simulink model "Playground"  (R2022a)
settings: Solver=VariableStepAuto  StartTime=0.0  StopTime=10.0  RelTol=1e-3
undefined symbols (not defined in the file): canChannel
libraries: canlib x4, canmsglib x2
settings Model: Creator=maxju  LastModifiedBy=maxju

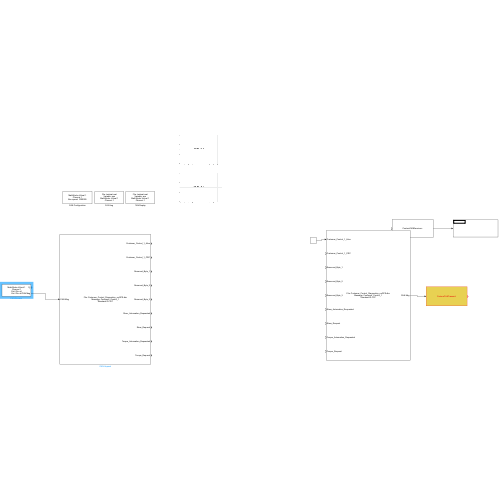
[thumbnail: Simulink's stored preview of the top-level diagram]
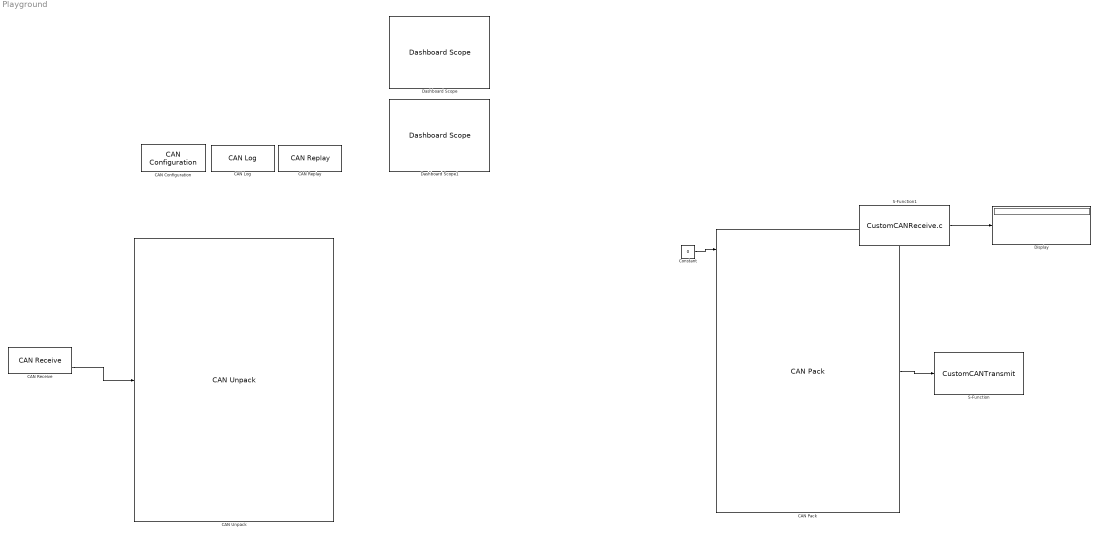
== system Playground ==
  CAN Configuration : canlib/CAN Configuration  BlockHandle=701.0001  Device=MathWorks Virtual 1 (Channel 1)  DeviceMenu=MathWorks Virtual 1 (Channel 1)  ObjConstructor=canChannel('MathWorks', 'Virtual 1', 1)  BusSpeed=1000000  EnableBitParameters=off  AckMode=Normal
      settings: SourceProductBaseCode=VN
  CAN Log : canlib/CAN Log  BlockHandle=706.0004  FullPathFileName=C:\Workspace\MATLAB Scripts\CAN_Blocks\testmat.mat  FileName=testmat.mat  VariableName=ans  MaxNumMessages=10000  LogFrom=CAN Bus  DeviceMenu=MathWorks Virtual 1 (Channel 1)  Device=MathWorks Virtual 1 (Channel 1)  ObjConstructor=canChannel('MathWorks', 'Virtual 1', 1)  SampleTime=0.01
      settings: SourceProductBaseCode=VN
  CAN Pack : canmsglib/CAN Pack  CANdbFile=C:\Workspace\XCU_eNV200_Shiftec\CAN\Customer_Control_Diagnostics_noGPS.dbc  MsgList=Customer_Control_1  MsgName=Customer_Control_1  MsgIDType=Standard (11-bit identifier)  MsgIdentifier=257  MsgLength=8  Remote=off  ApplyMinMax=off  BusOutput=off  SignalInfo={'Customer_Control_1_Alive','8','8','LE','unsigned','Standard','0','1','0','0','255';'Customer_Control_1_CRC','0','8','LE','unsigned','Standard','0','1','0','0','255';'Reserved_Byte_1','32','8','LE','unsigned','Standard','0','1','0','0','255';'Reserved_Byte_2','40','8','LE','unsigned','Standard','0','1','0','0','255';'Reserved_Byte_3','48','8','LE','unsigned','Standard','0','1','0','0','255';'Steer_Automation_Requested','56','1','LE','unsigned','Standard','0','1','0','0','1';'Steer_Request','16','8','LE','signed','Standard','0','1','0','-100','100';'Torque_Automation_Requested','60','1','LE','unsigned','Standard','0','1','0','0','1';'Torque_Request','24','8','LE','signed','Standard','0','1','0','-100','100'}
      settings: SourceProductBaseCode=XP,ME,VN  DataFormat=CANdb specified signals
  CAN Receive : canlib/CAN Receive  BlockHandle=702.0004  Device=MathWorks Virtual 1 (Channel 1)  DeviceMenu=MathWorks Virtual 1 (Channel 1)  ObjConstructor=canChannel('MathWorks', 'Virtual 1', 1)  EnableStandardIDsFilter=off  StdIDsCombo=Allow all  StandardIDs=0  EnableExtendedIDsFilter=off  ExtIDsCombo=Allow all  ExtendedIDs=0  SampleTime=0.01  MsgsPerTimestep=all  InternalFilterUpdateStatus=on  BusOutput=off
      settings: SourceProductBaseCode=VN
  CAN Replay : canlib/CAN Replay  BlockHandle=705.0002  FullPathFileName=C:\Workspace\MATLAB Scripts\CAN_Blocks\testmat.mat  FileName=testmat.mat  VariableName=ans  NoTimesReplay=Inf  ReplayTo=CAN Bus  DeviceMenu=MathWorks Virtual 1 (Channel 1)  Device=MathWorks Virtual 1 (Channel 1)  ObjConstructor=canChannel('MathWorks', 'Virtual 1', 1)  SampleTime=0.01  BusOutput=off
      settings: SourceProductBaseCode=VN
  CAN Unpack : canmsglib/CAN Unpack  CANdbFile=C:\Workspace\XCU_eNV200_Shiftec\CAN\Customer_Control_Diagnostics_noGPS.dbc  MsgList=Customer_Control_1  MsgName=Customer_Control_1  MsgIDType=Standard (11-bit identifier)  MsgIdentifier=257  MsgLength=8  SignalInfo={ 'Customer_Control_1_Alive', '8', '8', 'LE', 'unsigned', 'Standard', '0', '1', '0', '0', '255'; 'Customer_Control_1_CRC', '0', '8', 'LE', 'unsigned', 'Standard', '0', '1', '0', '0', '255'; 'Reserved_Byte_1', '32', '8', 'LE', 'unsigned', 'Standard', '0', '1', '0', '0', '255'; 'Reserved_Byte_2', '40', '8', 'LE', 'unsigned', 'Standard', '0', '1', '0', '0', '255'; 'Reserved_Byte_3', '48', '8', 'LE', 'unsigned', 'Standard', '0', '1', '0', '0', '255'; 'Steer_Automation_Requested', '56', '1', 'LE', 'unsigned', 'Standard', '0', '1', '0', '0', '1'; 'Steer_Request', '16', '8', 'LE', 'signed', 'Standard', '0', '1', '0', '-100', '100'; 'Torque_Automation_Requested', '60', '1', 'LE', 'unsigned', 'Standard', '0', '1', '0', '0', '1'; 'Torque_Request', '24', '8', 'LE', 'signed', 'Standard', '0', '1', '0', '-100', '100' }  IDPort=off  TimestampPort=off  ErrorPort=off  RemotePort=off  LengthPort=off  StatusPort=off  ApplyMinMax=off
      settings: SourceProductBaseCode=XP,ME,VN  DataFormat=CANdb specified signals
  Constant : Constant  Value=0
  Dashboard Scope : DashboardScope
  Dashboard Scope1 : DashboardScope
  Display : Display
  S-Function : S-Function  FunctionName=CustomCANTransmit  SFunctionDeploymentMode=off  EnableBusSupport=off
  S-Function1 : S-Function  FunctionName=CustomCANReceive.c  SFunctionDeploymentMode=off  EnableBusSupport=off
  wires:
  Constant/1 -> CAN Pack/1
  CAN Pack/1 -> S-Function/1
  S-Function1/1 -> Display/1
  CAN Receive/2 -> CAN Unpack/1
